simulink model "Clutch_TestBench"  (R2017a)
settings: Solver=FixedStepAuto  StartTime=0.0  StopTime=CycleTime  FixedStep=tloop  RelTol=1e-3
InitFcn:
  | clc
  | clear all;
  | CycleTime=49;
  | tloop=0.01;
undefined symbols (not defined in the file): clt, Clutch, Clutch2, Engine, lib_SystemDiag, SystemDiag
libraries: simulink x23, autolibcoupling x2
settings Model: Creator=Di Russo  LastModifiedBy=Di Russo

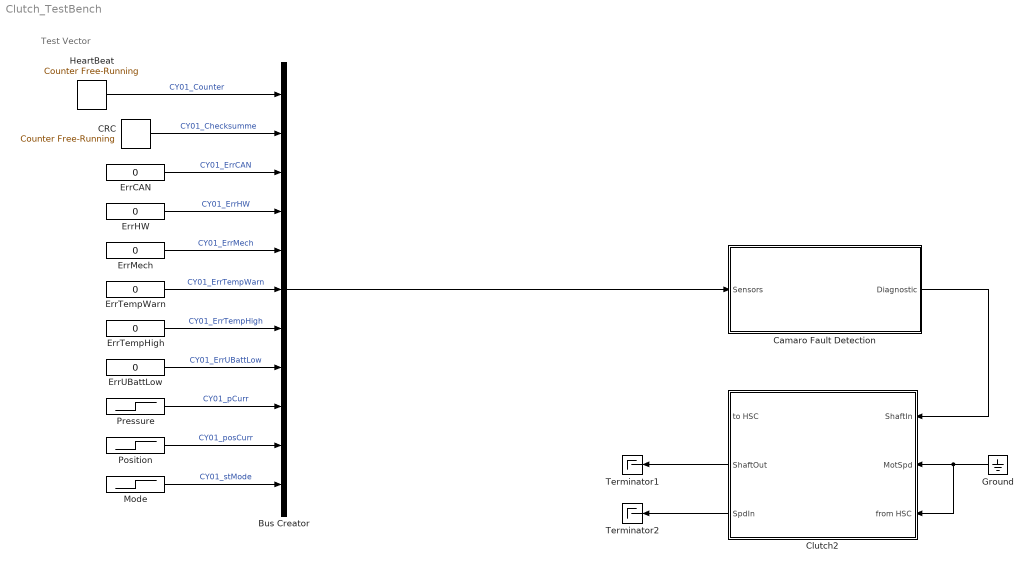
== system Clutch_TestBench ==
  note: Test Vector
  Bus Creator : BusCreator  Inputs=11
  "CRC " : simulink/Sources/Counter Free-Running  NumBits=16  tsamp=-1
  Camaro Fault Detection : Subsystem  AncestorBlock=lib_FaultDetection/Camaro Fault Detection
  Clutch2 : Subsystem  AncestorBlock=Clutch/Clutch2
      mask Display:
      | image('Images/Clutch.jpg')
      | color('red');
      | port_label('Input',1,'From HSC');
      | port_label('Input',2,'ShaftIn');
      | port_label('Input',3,'SpdOut');
      | port_label('Output',1,'To HSC');
      | port_label('Output',2,'ShaftOut');
      | port_label('Output',3,'SpdIn');
  ErrCAN : Constant  Value=0
  ErrHW : Constant  Value=0
  ErrMech : Constant  Value=0
  ErrTempHigh : Constant  Value=0
  ErrTempWarn : Constant  Value=0
  ErrUBattLow : Constant  Value=0
  Ground : Ground
  "HeartBeat " : simulink/Sources/Counter Free-Running  NumBits=4  tsamp=-1
  Mode : Step  After=7  SampleTime=0
  Position : Step  After=7000  SampleTime=0
  Pressure : Step  After=40  SampleTime=0
  Terminator1 : Terminator
  Terminator2 : Terminator
  wires:
  ErrCAN/1 -> Bus Creator/3  "CY01_ErrCAN"
  ErrTempWarn/1 -> Bus Creator/6  "CY01_ErrTempWarn"
  ErrTempHigh/1 -> Bus Creator/7  "CY01_ErrTempHigh"
  ErrUBattLow/1 -> Bus Creator/8  "CY01_ErrUBattLow"
  Pressure/1 -> Bus Creator/9  "CY01_pCurr"
  ErrMech/1 -> Bus Creator/5  "CY01_ErrMech"
  ErrHW/1 -> Bus Creator/4  "CY01_ErrHW"
  Mode/1 -> Bus Creator/11  "CY01_stMode"
  "HeartBeat "/1 -> Bus Creator/1  "CY01_Counter"
  Position/1 -> Bus Creator/10  "CY01_posCurr"
  Bus Creator/1 -> Camaro Fault Detection/1(Sensors)
  "CRC "/1 -> Bus Creator/2  "CY01_Checksumme"
  Camaro Fault Detection/1(Diagnostic) -> Clutch2/1(ShaftIn)
  Ground/1 -> Clutch2/3(from HSC), Clutch2/2(MotSpd)
  Clutch2/2(ShaftOut) -> Terminator1/1
  Clutch2/3(SpdIn) -> Terminator2/1

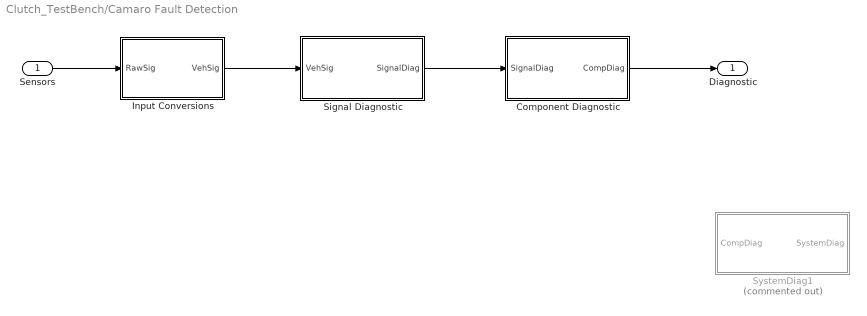
== system Clutch_TestBench/Camaro Fault Detection ==
  Sensors : Inport
  Component Diagnostic : Subsystem
  Input Conversions : Subsystem
  Signal Diagnostic : Subsystem
  SystemDiag1 : Subsystem  Commented=on  AncestorBlock=lib_SystemDiag/SystemDiag
  Diagnostic : Outport
  wires:
  Signal Diagnostic/1(SignalDiag) -> Component Diagnostic/1(SignalDiag)
  Component Diagnostic/1(CompDiag) -> Diagnostic/1
  Input Conversions/1(VehSig) -> Signal Diagnostic/1(VehSig)
  Sensors/1 -> Input Conversions/1(RawSig)

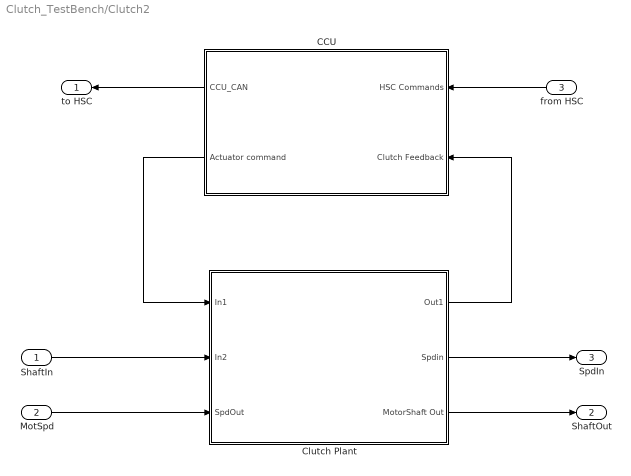
== system Clutch_TestBench/Clutch2 ==
  ShaftIn : Inport
  MotSpd : Inport  Port=2
  from HSC : Inport  Port=3
  CCU : Subsystem
      mask Display: image('SoftECU.jpg')
  Clutch Plant : Subsystem
      mask Display:
      | image('Images/Clutch.jpg')
      | color('red');
      | port_label('Input',2,'ShaftIn');
      | port_label('Input',3,'SpdOut');
      | port_label('Output',3,'ShaftOut');
      | port_label('Output',2,'SpdIn');
  to HSC : Outport
  ShaftOut : Outport  Port=2
  SpdIn : Outport  Port=3
  wires:
  Clutch Plant/1(Out1) -> CCU/2(Clutch Feedback)
  CCU/1("CCU_CAN ") -> to HSC/1
  Clutch Plant/3(MotorShaft Out) -> ShaftOut/1
  Clutch Plant/2(Spdin) -> SpdIn/1
  MotSpd/1 -> Clutch Plant/3(SpdOut)
  ShaftIn/1 -> Clutch Plant/2(In2)
  CCU/2("Actuator command ") -> Clutch Plant/1(In1)
  from HSC/1 -> CCU/1(HSC Commands)

== system Clutch_TestBench/Camaro Fault Detection/Component Diagnostic ==
  note: Component Status Setting Rule
      | xxx_CompStatus could be 0, 1, 2 or 3
      | 0: component needs to be offline
      | 1: component needs torque plant to deliver creep torque
      | 2: component needs torque plant to limit maximum torque delivery
      | 3: component needs torque plant to operate normally
  note: Component Diagnostics
  SignalDiag : Inport
  Clutch Component Diagnostic : Subsystem
  Override Clutch Status : Subsystem
  CompDiag : Outport
  wires:
  Clutch Component Diagnostic/1(Out1) -> Override Clutch Status/1(In1)  "CCM_CompDiag"
  Override Clutch Status/1(Out1) -> CompDiag/1  "Clutch_Status"
  SignalDiag/1 -> Clutch Component Diagnostic/1(In1)  "RawSig"

== system Clutch_TestBench/Camaro Fault Detection/Input Conversions ==
  note: Input Conversions and Override Switches
  note: These subsystems convert variable types to match those used in the
      | supervisor. In addition, override switches installed on each signal can
      | be used to manually override and signal for testing purposes
  RawSig : Inport
  Clutch_Conversions : Subsystem
  VehSig : Outport
  wires:
  Clutch_Conversions/1(Out1) -> VehSig/1
  RawSig/1 -> Clutch_Conversions/1(Sensors)  "RawSig"

== system Clutch_TestBench/Camaro Fault Detection/Signal Diagnostic ==
  note: These subsystems evaluate each signal for proper value range and other checks
  note: Signal Diagnostics
  VehSig : Inport
  Clutch Signal Diagnostic : Subsystem
  Subsystem1 : Subsystem
      mask Display: fprintf('Signal Naming Rule')
  SignalDiag : Outport
  wires:
  Clutch Signal Diagnostic/1(Out2) -> SignalDiag/1  "Clutch_SigDiag"
  VehSig/1 -> Clutch Signal Diagnostic/1(Sensors1)

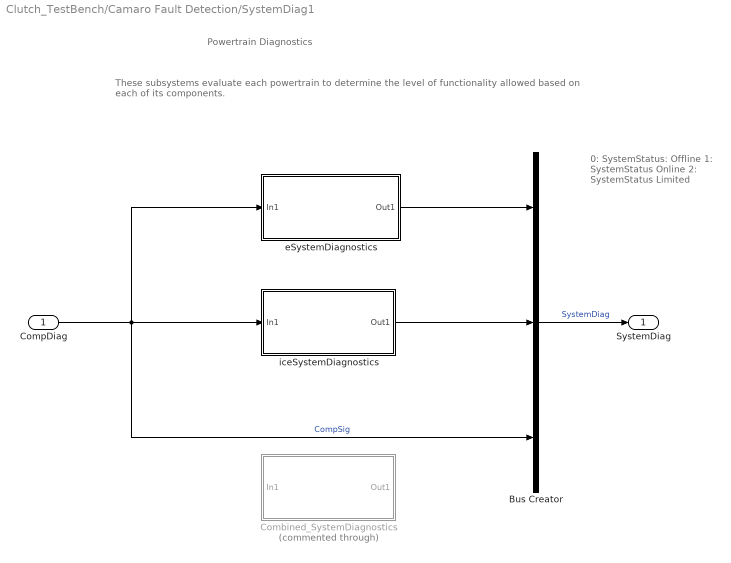
== system Clutch_TestBench/Camaro Fault Detection/SystemDiag1 ==
  note: 0: SystemStatus: Offline
      | 1: SystemStatus Online
      | 2: SystemStatus Limited
  note: Powertrain Diagnostics
  note: These subsystems evaluate each powertrain to determine
      | the level of functionality allowed based on each of its components.
  CompDiag : Inport
  Bus Creator : BusCreator  Inputs=3
  Combined_SystemDiagnostics : Subsystem  Commented=through
  eSystemDiagnostics : Subsystem
  iceSystemDiagnostics : Subsystem
  SystemDiag : Outport
  wires:
  eSystemDiagnostics/1(Out1) -> Bus Creator/1
  Bus Creator/1 -> SystemDiag/1  "SystemDiag"
  CompDiag/1 -> iceSystemDiagnostics/1(In1), Bus Creator/3, eSystemDiagnostics/1(In1)  "CompSig"
  iceSystemDiagnostics/1(Out1) -> Bus Creator/2

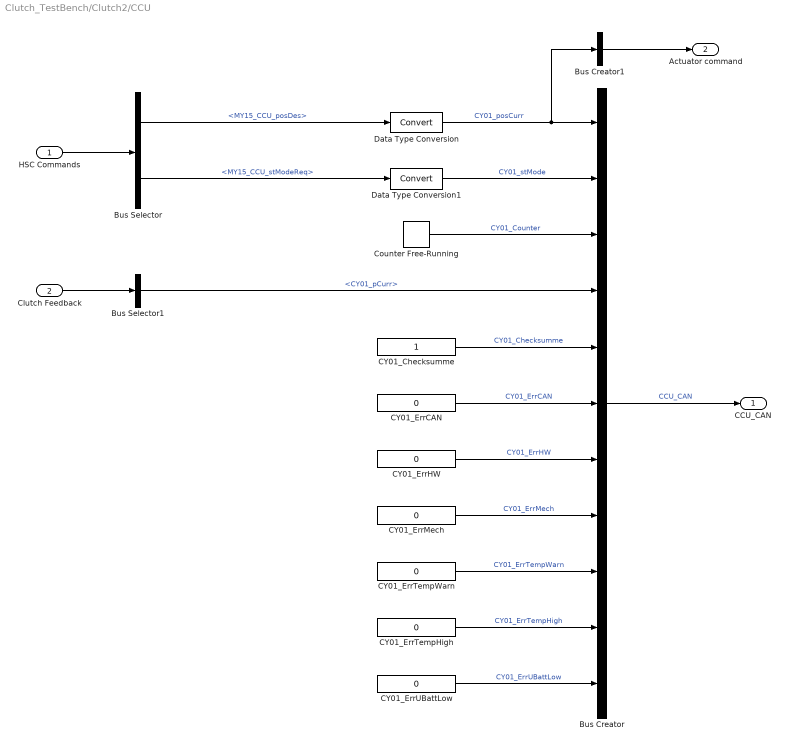
== system Clutch_TestBench/Clutch2/CCU ==
  HSC Commands : Inport
  Clutch Feedback : Inport  Port=2
  Bus Creator : BusCreator  Inputs=11
  Bus Creator1 : BusCreator  Inputs=1
  Bus Selector : BusSelector  OutputSignals=MY15_CCU_posDes,MY15_CCU_stModeReq
  Bus Selector1 : BusSelector  OutputSignals=CY01_pCurr
  CY01_Checksumme : Constant
  CY01_ErrCAN : Constant  Value=0
  CY01_ErrHW : Constant  Value=0
  CY01_ErrMech : Constant  Value=0
  CY01_ErrTempHigh : Constant  Value=0
  CY01_ErrTempWarn : Constant  Value=0
  CY01_ErrUBattLow : Constant  Value=0
  Counter Free-Running : simulink/Sources/Counter Free-Running  NumBits=15  tsamp=-1
  Data Type Conversion : DataTypeConversion
  Data Type Conversion1 : DataTypeConversion
  "CCU_CAN " : Outport
  "Actuator command " : Outport  Port=2
  wires:
  Clutch Feedback/1 -> Bus Selector1/1
  Data Type Conversion1/1 -> Bus Creator/2  "CY01_stMode"
  Bus Selector/2 -> Data Type Conversion1/1  "<MY15_CCU_stModeReq>"
  Counter Free-Running/1 -> Bus Creator/3  "CY01_Counter"
  Bus Creator1/1 -> "Actuator command "/1
  Bus Creator/1 -> "CCU_CAN "/1  "CCU_CAN"
  Data Type Conversion/1 -> Bus Creator1/1, Bus Creator/1  "CY01_posCurr"
  Bus Selector/1 -> Data Type Conversion/1  "<MY15_CCU_posDes>"
  HSC Commands/1 -> Bus Selector/1
  Bus Selector1/1 -> Bus Creator/4  "<CY01_pCurr>"
  CY01_Checksumme/1 -> Bus Creator/5  "CY01_Checksumme"
  CY01_ErrCAN/1 -> Bus Creator/6  "CY01_ErrCAN"
  CY01_ErrHW/1 -> Bus Creator/7  "CY01_ErrHW"
  CY01_ErrMech/1 -> Bus Creator/8  "CY01_ErrMech"
  CY01_ErrUBattLow/1 -> Bus Creator/11  "CY01_ErrUBattLow"
  CY01_ErrTempHigh/1 -> Bus Creator/10  "CY01_ErrTempHigh"
  CY01_ErrTempWarn/1 -> Bus Creator/9  "CY01_ErrTempWarn"

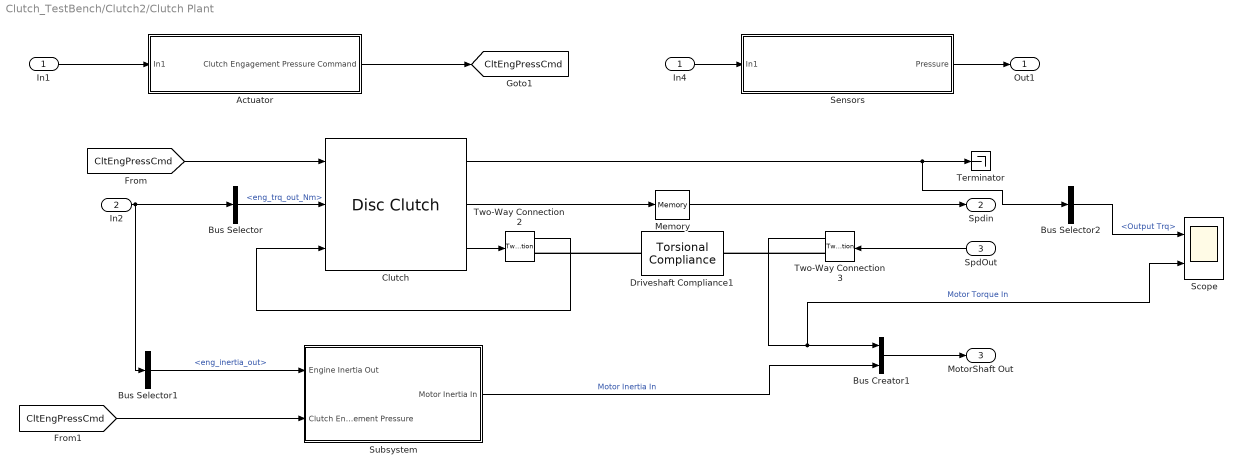
== system Clutch_TestBench/Clutch2/Clutch Plant ==
  In1 : Inport
  In2 : Inport  Port=2
  SpdOut : Inport  Port=3
  " Actuator" : Subsystem
  " Sensors " : Subsystem
  Bus Creator1 : BusCreator  Inputs=2
  Bus Selector : BusSelector  OutputSignals=eng_trq_out_Nm
  Bus Selector1 : BusSelector  OutputSignals=eng_inertia_out
  Bus Selector2 : BusSelector  OutputSignals=Output.Output Trq
  Clutch : autolibcoupling/Disc Clutch  port_config=Simulink  Reff=0.121  Ndisk=1  Aeff=0.02129  Jin=Engine.Inertia + (0.75*clt.plant.init.inertia)  Jout=.1 + (0.25*clt.plant.init.inertia)  muk=0.25  mus=0.3  bin=.001*2  bout=.001*2  win_o=0  wout_o=0  tauC=0.01*10  InitiallyLocked=on  maxAbsSpd=3000  blkID=1
      settings: SourceProductName=Powertrain Blockset  SourceProductBaseCode=PW
  Driveshaft Compliance1 : autolibcoupling/Torsional Compliance  port_config=Two-way connection  k=1000000  b=100  theta_o=0  domega_o=0  omega_c=100  blkID=0
      settings: SourceProductName=Powertrain Blockset
  In4 : InportShadow
  Memory : Memory
  Scope : Scope  NumInputPorts=2
  Subsystem : Subsystem
  Terminator : Terminator
  Two-Way Connection2 : TwoWayConnection
  Two-Way Connection3 : TwoWayConnection
  Out1 : Outport
  Spdin : Outport  Port=2
  MotorShaft Out : Outport  Port=3
  tag scope: CltEngPressCmd=global
  wires:
  " Sensors "/1(Pressure) -> Out1/1
  In4/1 -> " Sensors "/1(In1)
  Bus Selector/1 -> Clutch/2  "<eng_trq_out_Nm>"
  [CltEngPressCmd] -> Clutch/1
  " Actuator"/1(Clutch Engagement Pressure Command) -> [CltEngPressCmd]
  Clutch/1 -> Bus Selector2/1, Terminator/1
  In1/1 -> " Actuator"/1(In1)
  Clutch/3 -> Two-Way Connection2/1
  SpdOut/1 -> Two-Way Connection3/1
  In2/1 -> Bus Selector1/1, Bus Selector/1
  Memory/1 -> Spdin/1
  Two-Way Connection2/1 -> Clutch/3
  Two-Way Connection3/1 -> Scope/2, Bus Creator1/1  "Motor Torque In"
  Clutch/2 -> Memory/1
  [CltEngPressCmd] -> Subsystem/2(Clutch Engagement Pressure)
  Bus Selector1/1 -> Subsystem/1(Engine Inertia Out)  "<eng_inertia_out>"
  Bus Creator1/1 -> MotorShaft Out/1
  Subsystem/1(Motor Inertia In) -> Bus Creator1/2  "Motor Inertia In"
  Bus Selector2/1 -> Scope/1  "<Output Trq>"
  connections:
  Driveshaft Compliance1/LConn1 -- Two-Way Connection2/RConn1
  Two-Way Connection3/RConn1 -- Driveshaft Compliance1/RConn1

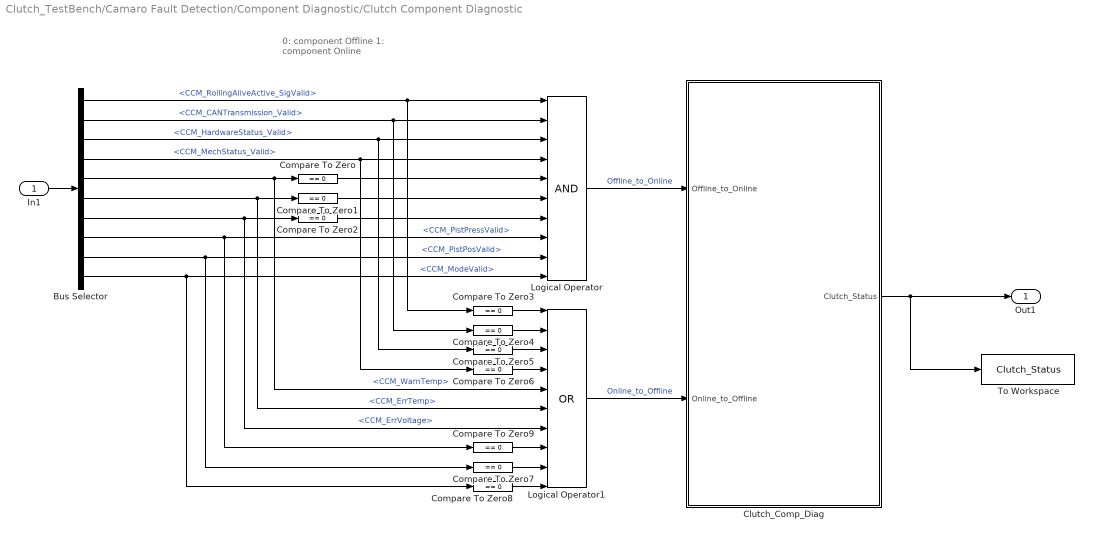
== system Clutch_TestBench/Camaro Fault Detection/Component Diagnostic/Clutch Component Diagnostic ==
  note: 0: component Offline
      | 1: component Online
  In1 : Inport
  Bus Selector : BusSelector  OutputSignals=CCM_RollingAliveActive_SigValid,CCM_CANTransmission_Valid,CCM_HardwareStatus_Valid,CCM_MechStatus_Valid,CCM_WarnTemp,CCM_ErrTemp,CCM_ErrVoltage,CCM_PistPressValid,CCM_PistPosValid,CCM_ModeValid
  Clutch_Comp_Diag : Stateflow chart  TreatAsAtomicUnit=on
  Compare To Zero{,1..9} (10 alike) : simulink/Logic and Bit Operations/Compare To Zero  relop===  OutDataTypeStr=boolean
  Logical Operator : Logic  Inputs=10  AllPortsSameDT=off  OutDataTypeStr=boolean
  Logical Operator1 : Logic  Operator=OR  Inputs=10  AllPortsSameDT=off  OutDataTypeStr=boolean
  To Workspace : ToWorkspace  VariableName=Clutch_Status  SampleTime=-1
  Out1 : Outport
  wires:
  In1/1 -> Bus Selector/1
  Bus Selector/1 -> Compare To Zero3/1, Logical Operator/1  "<CCM_RollingAliveActive_SigValid>"
  Bus Selector/2 -> Compare To Zero4/1, Logical Operator/2  "<CCM_CANTransmission_Valid>"
  Bus Selector/3 -> Compare To Zero5/1, Logical Operator/3  "<CCM_HardwareStatus_Valid>"
  Bus Selector/4 -> Compare To Zero6/1, Logical Operator/4  "<CCM_MechStatus_Valid>"
  Bus Selector/5 -> Logical Operator1/5, Compare To Zero/1  "<CCM_WarnTemp>"
  Bus Selector/6 -> Logical Operator1/6, Compare To Zero1/1  "<CCM_ErrTemp>"
  Bus Selector/7 -> Logical Operator1/7, Compare To Zero2/1  "<CCM_ErrVoltage>"
  Bus Selector/8 -> Compare To Zero9/1, Logical Operator/8  "<CCM_PistPressValid>"
  Bus Selector/9 -> Compare To Zero7/1, Logical Operator/9  "<CCM_PistPosValid>"
  Bus Selector/10 -> Compare To Zero8/1, Logical Operator/10  "<CCM_ModeValid>"
  Logical Operator/1 -> Clutch_Comp_Diag/1(Offline_to_Online)  "Offline_to_Online"
  Logical Operator1/1 -> Clutch_Comp_Diag/2(Online_to_Offline)  "Online_to_Offline"
  Clutch_Comp_Diag/1(Clutch_Status) -> To Workspace/1, Out1/1
  Compare To Zero/1 -> Logical Operator/5
  Compare To Zero1/1 -> Logical Operator/6
  Compare To Zero2/1 -> Logical Operator/7
  Compare To Zero3/1 -> Logical Operator1/1
  Compare To Zero4/1 -> Logical Operator1/2
  Compare To Zero5/1 -> Logical Operator1/3
  Compare To Zero6/1 -> Logical Operator1/4
  Compare To Zero7/1 -> Logical Operator1/9
  Compare To Zero8/1 -> Logical Operator1/10
  Compare To Zero9/1 -> Logical Operator1/8

== system Clutch_TestBench/Camaro Fault Detection/Component Diagnostic/Override Clutch Status ==
  note: This subsystem is used to override the model value of a signal to a constant value
  note: Override Switch Subsystem
  In1 : Inport
  Multiport Switch : MultiPortSwitch  DataPortOrder=Zero-based contiguous  Inputs=2  zeroidx=on
  Override Value : Constant  Value=2  OutDataTypeStr=double
  Signal Override Switch 0 = Use Model 1 = Use Constant : Constant  Value=0
  Out1 : Outport
  wires:
  Signal Override Switch 0 = Use Model 1 = Use Constant/1 -> Multiport Switch/1
  In1/1 -> Multiport Switch/2
  Multiport Switch/1 -> Out1/1
  Override Value/1 -> Multiport Switch/3

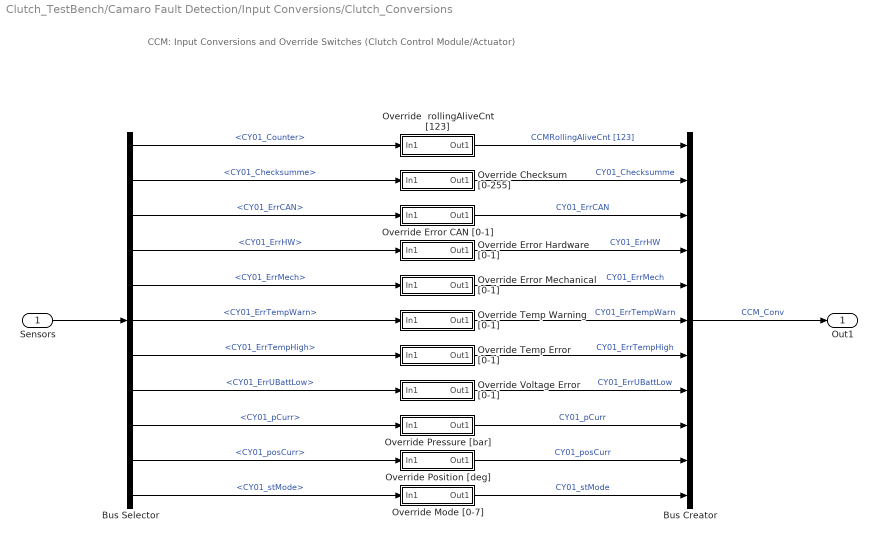
== system Clutch_TestBench/Camaro Fault Detection/Input Conversions/Clutch_Conversions ==
  note: CCM: Input Conversions and Override Switches
      | (Clutch Control Module/Actuator)
  Sensors : Inport
  Bus Creator : BusCreator  Inputs=11
  Bus Selector : BusSelector  OutputSignals=CY01_Counter,CY01_Checksumme,CY01_ErrCAN,CY01_ErrHW,CY01_ErrMech,CY01_ErrTempWarn,CY01_ErrTempHigh,CY01_ErrUBattLow,CY01_pCurr,CY01_posCurr,CY01_stMode
  Override  rollingAliveCnt [123] : Subsystem
  Override Checksum [0-255] : Subsystem
  Override Error CAN [0-1] : Subsystem
  Override Error Hardware [0-1] : Subsystem
  Override Error Mechanical [0-1] : Subsystem
  Override Mode [0-7] : Subsystem
  Override Position [deg] : Subsystem
  Override Pressure [bar] : Subsystem
  Override Temp Error [0-1] : Subsystem
  Override Temp Warning [0-1] : Subsystem
  Override Voltage Error [0-1] : Subsystem
  Out1 : Outport
  wires:
  Override Mode [0-7]/1(Out1) -> Bus Creator/11  "CY01_stMode"
  Override Position [deg]/1(Out1) -> Bus Creator/10  "CY01_posCurr"
  Override Pressure [bar]/1(Out1) -> Bus Creator/9  "CY01_pCurr"
  Bus Selector/11 -> Override Mode [0-7]/1(In1)  "<CY01_stMode>"
  Bus Selector/10 -> Override Position [deg]/1(In1)  "<CY01_posCurr>"
  Bus Selector/9 -> Override Pressure [bar]/1(In1)  "<CY01_pCurr>"
  Override Voltage Error [0-1]/1(Out1) -> Bus Creator/8  "CY01_ErrUBattLow"
  Override Temp Error [0-1]/1(Out1) -> Bus Creator/7  "CY01_ErrTempHigh"
  Override Temp Warning [0-1]/1(Out1) -> Bus Creator/6  "CY01_ErrTempWarn"
  Override Error Mechanical [0-1]/1(Out1) -> Bus Creator/5  "CY01_ErrMech"
  Override Error Hardware [0-1]/1(Out1) -> Bus Creator/4  "CY01_ErrHW"
  Override Error CAN [0-1]/1(Out1) -> Bus Creator/3  "CY01_ErrCAN"
  Override Checksum [0-255]/1(Out1) -> Bus Creator/2  "CY01_Checksumme"
  Bus Selector/8 -> Override Voltage Error [0-1]/1(In1)  "<CY01_ErrUBattLow>"
  Bus Selector/7 -> Override Temp Error [0-1]/1(In1)  "<CY01_ErrTempHigh>"
  Bus Selector/6 -> Override Temp Warning [0-1]/1(In1)  "<CY01_ErrTempWarn>"
  Bus Selector/5 -> Override Error Mechanical [0-1]/1(In1)  "<CY01_ErrMech>"
  Bus Selector/4 -> Override Error Hardware [0-1]/1(In1)  "<CY01_ErrHW>"
  Bus Selector/3 -> Override Error CAN [0-1]/1(In1)  "<CY01_ErrCAN>"
  Bus Selector/2 -> Override Checksum [0-255]/1(In1)  "<CY01_Checksumme>"
  Sensors/1 -> Bus Selector/1
  Bus Selector/1 -> Override  rollingAliveCnt [123]/1(In1)  "<CY01_Counter>"
  Override  rollingAliveCnt [123]/1(Out1) -> Bus Creator/1  "CCMRollingAliveCnt [123]"
  Bus Creator/1 -> Out1/1  "CCM_Conv"

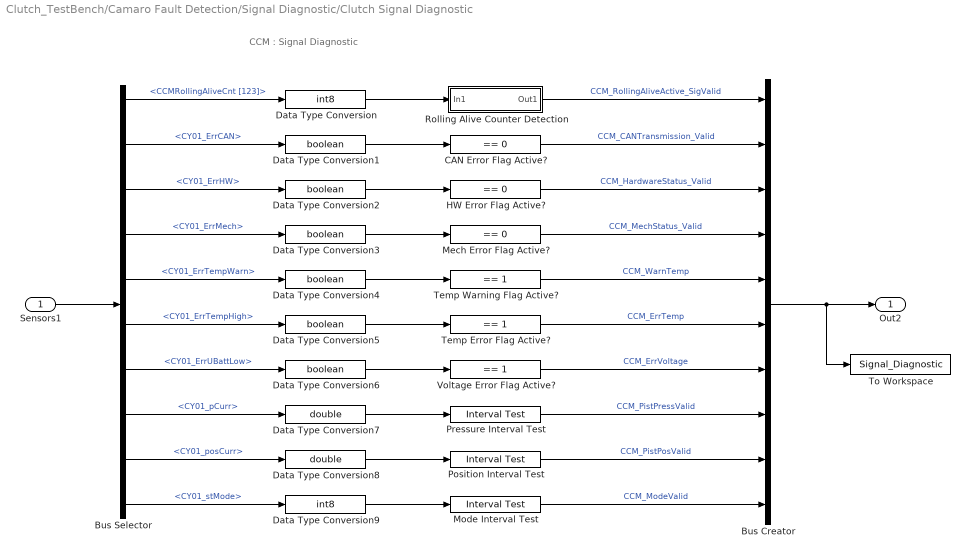
== system Clutch_TestBench/Camaro Fault Detection/Signal Diagnostic/Clutch Signal Diagnostic ==
  note: CCM : Signal Diagnostic
  Sensors1 : Inport
  Bus Creator : BusCreator  Inputs=10
  Bus Selector : BusSelector  OutputSignals=CCMRollingAliveCnt [123],CY01_ErrCAN,CY01_ErrHW,CY01_ErrMech,CY01_ErrTempWarn,CY01_ErrTempHigh,CY01_ErrUBattLow,CY01_pCurr,CY01_posCurr,CY01_stMode
  CAN Error Flag Active? : simulink/Logic and Bit Operations/Compare To Constant  relop===  const=0  OutDataTypeStr=boolean
  Data Type Conversion : DataTypeConversion  OutDataTypeStr=int8
  Data Type Conversion{1..6} (6 alike) : DataTypeConversion  OutDataTypeStr=boolean
  Data Type Conversion7 : DataTypeConversion  OutDataTypeStr=double
  Data Type Conversion8 : DataTypeConversion  OutDataTypeStr=double
  Data Type Conversion9 : DataTypeConversion  OutDataTypeStr=int8
  HW Error Flag Active? : simulink/Logic and Bit Operations/Compare To Constant  relop===  const=0  OutDataTypeStr=boolean
  Mech Error Flag Active? : simulink/Logic and Bit Operations/Compare To Constant  relop===  const=0  OutDataTypeStr=boolean
  Mode Interval Test : simulink/Logic and Bit Operations/Interval Test  IntervalClosedRight=on  uplimit=7  IntervalClosedLeft=on  lowlimit=0  OutDataTypeStr=boolean
  Position Interval Test : simulink/Logic and Bit Operations/Interval Test  IntervalClosedRight=on  uplimit=8190  IntervalClosedLeft=on  lowlimit=0  OutDataTypeStr=boolean
  Pressure Interval Test : simulink/Logic and Bit Operations/Interval Test  IntervalClosedRight=on  uplimit=50.6  IntervalClosedLeft=on  lowlimit=0  OutDataTypeStr=boolean
  Rolling Alive Counter Detection : Subsystem
  Temp Error Flag Active? : simulink/Logic and Bit Operations/Compare To Constant  relop===  const=1  OutDataTypeStr=boolean
  Temp Warning Flag Active? : simulink/Logic and Bit Operations/Compare To Constant  relop===  const=1  OutDataTypeStr=boolean
  To Workspace : ToWorkspace  VariableName=Signal_Diagnostic  SampleTime=-1
  Voltage Error Flag Active? : simulink/Logic and Bit Operations/Compare To Constant  relop===  const=1  OutDataTypeStr=boolean
  Out2 : Outport
  wires:
  Mode Interval Test/1 -> Bus Creator/10  "CCM_ModeValid"
  Bus Selector/10 -> Data Type Conversion9/1  "<CY01_stMode>"
  Position Interval Test/1 -> Bus Creator/9  "CCM_PistPosValid"
  Bus Selector/9 -> Data Type Conversion8/1  "<CY01_posCurr>"
  Pressure Interval Test/1 -> Bus Creator/8  "CCM_PistPressValid"
  Bus Selector/8 -> Data Type Conversion7/1  "<CY01_pCurr>"
  Voltage Error Flag Active?/1 -> Bus Creator/7  "CCM_ErrVoltage"
  Bus Selector/7 -> Data Type Conversion6/1  "<CY01_ErrUBattLow>"
  Temp Error Flag Active?/1 -> Bus Creator/6  "CCM_ErrTemp"
  Bus Selector/6 -> Data Type Conversion5/1  "<CY01_ErrTempHigh>"
  Temp Warning Flag Active?/1 -> Bus Creator/5  "CCM_WarnTemp"
  Bus Selector/5 -> Data Type Conversion4/1  "<CY01_ErrTempWarn>"
  Mech Error Flag Active?/1 -> Bus Creator/4  "CCM_MechStatus_Valid"
  Bus Selector/4 -> Data Type Conversion3/1  "<CY01_ErrMech>"
  HW Error Flag Active?/1 -> Bus Creator/3  "CCM_HardwareStatus_Valid"
  Bus Selector/3 -> Data Type Conversion2/1  "<CY01_ErrHW>"
  CAN Error Flag Active?/1 -> Bus Creator/2  "CCM_CANTransmission_Valid"
  Bus Selector/2 -> Data Type Conversion1/1  "<CY01_ErrCAN>"
  Rolling Alive Counter Detection/1(Out1) -> Bus Creator/1  "CCM_RollingAliveActive_SigValid"
  Bus Selector/1 -> Data Type Conversion/1  "<CCMRollingAliveCnt [123]>"
  Bus Creator/1 -> To Workspace/1, Out2/1
  Sensors1/1 -> Bus Selector/1
  Data Type Conversion/1 -> Rolling Alive Counter Detection/1(In1)
  Data Type Conversion1/1 -> CAN Error Flag Active?/1
  Data Type Conversion2/1 -> HW Error Flag Active?/1
  Data Type Conversion3/1 -> Mech Error Flag Active?/1
  Data Type Conversion4/1 -> Temp Warning Flag Active?/1
  Data Type Conversion5/1 -> Temp Error Flag Active?/1
  Data Type Conversion6/1 -> Voltage Error Flag Active?/1
  Data Type Conversion7/1 -> Pressure Interval Test/1
  Data Type Conversion8/1 -> Position Interval Test/1
  Data Type Conversion9/1 -> Mode Interval Test/1

== system Clutch_TestBench/Camaro Fault Detection/Signal Diagnostic/Subsystem1 ==
  note: Signal Valid Setting Rule
      | xxx_yyy_[z]_SigValid could be 0 or 1
      | 0: signal invalid
      | 1: signal vaild
  note: Signal Naming Rule
      | Example: xxx_yyy_[z]_SigValid
      | xxx: source of the signal (Drv, Clu, BCM, ECM, TCM, BMS and MCU)
      | yyy: description of the signal
      | z: unit of the signal (V, A, Nm, m/s, %, 01, 0123, etc.)

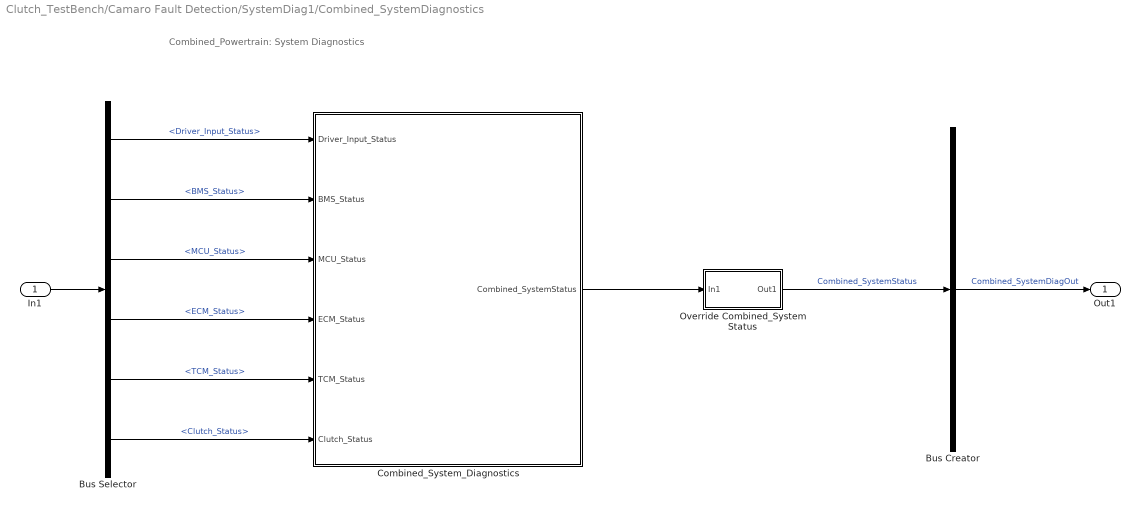
== system Clutch_TestBench/Camaro Fault Detection/SystemDiag1/Combined_SystemDiagnostics ==
  note: Combined_Powertrain: System Diagnostics
  In1 : Inport
  Bus Creator : BusCreator  Inputs=1
  Bus Selector : BusSelector  OutputSignals=Driver_Input_Status.Driver_Input_Status,BMS_Status.BMS_Status,MCU_Status.MCU_Status,ECM_Status.ECM_Status,TCM_CompDiag.TCM_Status,Clutch_Status.Clutch_Status
  Combined_System_Diagnostics : Stateflow chart  TreatAsAtomicUnit=on
  Override Combined_System Status : Subsystem
  Out1 : Outport
  wires:
  In1/1 -> Bus Selector/1
  Bus Creator/1 -> Out1/1  "Combined_SystemDiagOut"
  Override Combined_System Status/1(Out1) -> Bus Creator/1  "Combined_SystemStatus"
  Bus Selector/1 -> Combined_System_Diagnostics/1(Driver_Input_Status)  "<Driver_Input_Status>"
  Bus Selector/2 -> Combined_System_Diagnostics/2(BMS_Status)  "<BMS_Status>"
  Bus Selector/3 -> Combined_System_Diagnostics/3(MCU_Status)  "<MCU_Status>"
  Bus Selector/4 -> Combined_System_Diagnostics/4(ECM_Status)  "<ECM_Status>"
  Bus Selector/5 -> Combined_System_Diagnostics/5(TCM_Status)  "<TCM_Status>"
  Bus Selector/6 -> Combined_System_Diagnostics/6(Clutch_Status)  "<Clutch_Status>"
  Combined_System_Diagnostics/1(Combined_SystemStatus) -> Override Combined_System Status/1(In1)

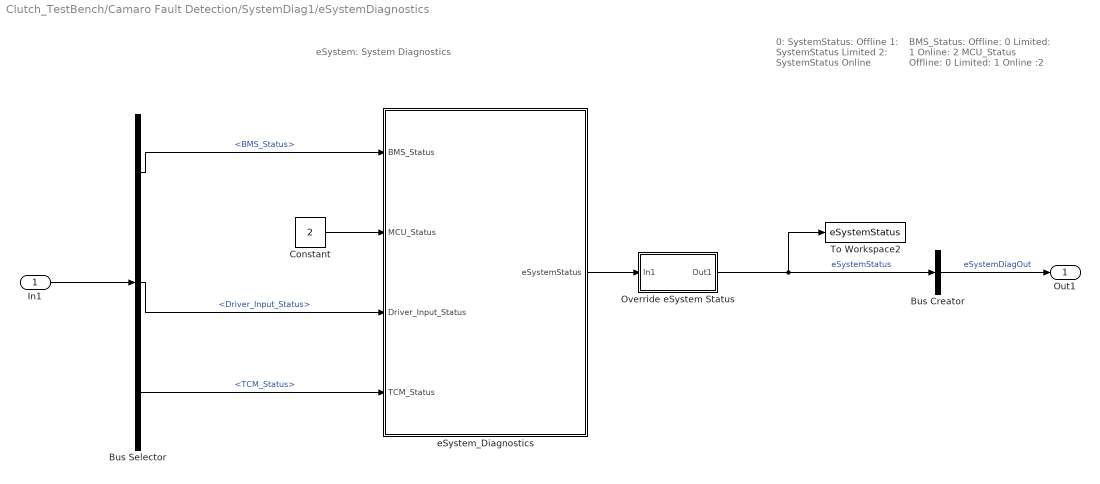
== system Clutch_TestBench/Camaro Fault Detection/SystemDiag1/eSystemDiagnostics ==
  note: BMS_Status:
      | Offline: 0
      | Limited: 1
      | Online: 2
      |
      | MCU_Status
      | Offline: 0
      | Limited: 1
      | Online :2
  note: 0: SystemStatus: Offline
      | 1: SystemStatus Limited
      | 2: SystemStatus Online
  note: eSystem: System Diagnostics
  In1 : Inport
  Bus Creator : BusCreator  Inputs=1
  Bus Selector : BusSelector  OutputSignals=BMS_Status,Driver_Input_Status,TCM_Status
  Constant : Constant  Value=2
  Override eSystem Status : Subsystem
  To Workspace2 : ToWorkspace  VariableName=eSystemStatus  SaveFormat=Timeseries  SampleTime=-1
  eSystem_Diagnostics : Stateflow chart  TreatAsAtomicUnit=on
  Out1 : Outport
  wires:
  Constant/1 -> eSystem_Diagnostics/2(MCU_Status)
  In1/1 -> Bus Selector/1
  Bus Selector/1 -> eSystem_Diagnostics/1(BMS_Status)  "<BMS_Status>"
  Bus Creator/1 -> Out1/1  "eSystemDiagOut"
  Bus Selector/2 -> eSystem_Diagnostics/3(Driver_Input_Status)  "<Driver_Input_Status>"
  Override eSystem Status/1(Out1) -> To Workspace2/1, Bus Creator/1  "eSystemStatus"
  eSystem_Diagnostics/1(eSystemStatus) -> Override eSystem Status/1(In1)
  Bus Selector/3 -> eSystem_Diagnostics/4(TCM_Status)  "<TCM_Status>"

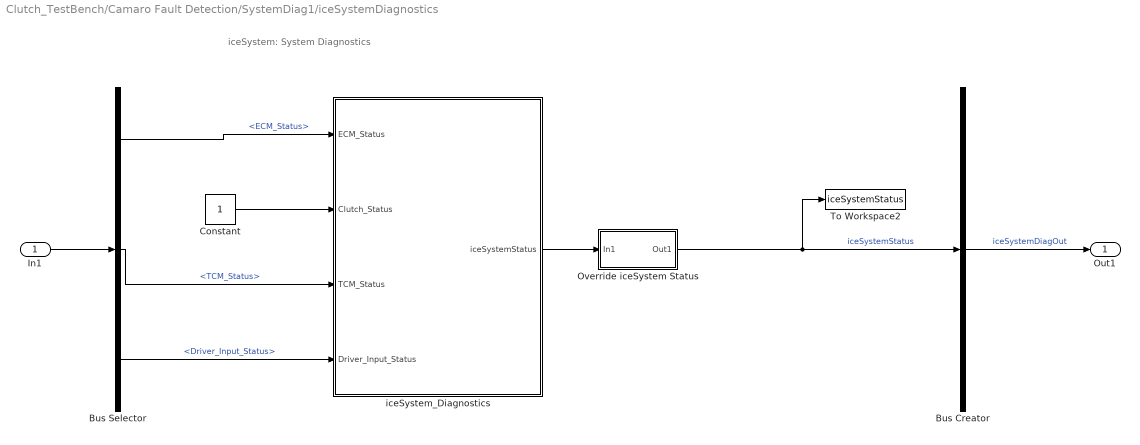
== system Clutch_TestBench/Camaro Fault Detection/SystemDiag1/iceSystemDiagnostics ==
  note: iceSystem: System Diagnostics
  In1 : Inport
  Bus Creator : BusCreator  Inputs=1
  Bus Selector : BusSelector  OutputSignals=ECM_Status,TCM_Status,Driver_Input_Status
  Constant : Constant
  Override iceSystem Status : Subsystem
  To Workspace2 : ToWorkspace  VariableName=iceSystemStatus  SaveFormat=Timeseries  SampleTime=-1
  iceSystem_Diagnostics : Stateflow chart  TreatAsAtomicUnit=on
  Out1 : Outport
  wires:
  Override iceSystem Status/1(Out1) -> To Workspace2/1, Bus Creator/1  "iceSystemStatus"
  Bus Selector/1 -> iceSystem_Diagnostics/1(ECM_Status)  "<ECM_Status>"
  Bus Creator/1 -> Out1/1  "iceSystemDiagOut"
  In1/1 -> Bus Selector/1
  Bus Selector/2 -> iceSystem_Diagnostics/3(TCM_Status)  "<TCM_Status>"
  Bus Selector/3 -> iceSystem_Diagnostics/4(Driver_Input_Status)  "<Driver_Input_Status>"
  iceSystem_Diagnostics/1(iceSystemStatus) -> Override iceSystem Status/1(In1)
  Constant/1 -> iceSystem_Diagnostics/2(Clutch_Status)

== system Clutch_TestBench/Clutch2/Clutch Plant/ Actuator ==
  In1 : Inport
  Actuator Position to Clutch Engagement Pressure : Lookup_n-D  NumberOfTableDimensions=1  BreakpointsForDimension1=|  Table=|  InternalRulePriority=Speed  RndMeth=Simplest  InputSameDT=on
      BreakpointsForDimension1=|
      | [0
      | 100
      | 200
      | 300
      | 400
      | 500
      | 600
      | 700
      | 800
      | 900
      | 1000
      | 1100
      | 1200
      | 1300
      | 1400
      | 1500
      | 1600
      | 1700
      | 1800
      | 1900
      | 2000
      | 2100
      | 2200
      | 2300
      | 2400
      | 2500
      | 2600
      | 2700
      | 2800
      | 2900
      | 3000
      | 3100
      | 3200
      | 3300
      | 3400
      | 3500
      | 3600
      | 3700
      | 3800
      | 3900
      | 4000
      | 4100
      | 4200
      | 4300
      | 4400
      | 4500
      | 4600
      | 4700
      | 4800
      | 4900
      | 5000
      | 5100
      | 5200
      | 5300
      | 5400
      | 5500
      | 5600
      | 5700
      | 5800
      | 5900
      | 6000
      | 6100
      | 6200
      | 6300
      | 6400
      | 
      | ]
      Table=|
      | [892800
      | 892800
      | 892800
      | 833280
      | 773760
      | 714240
      | 654720
      | 595200
      | 535680
      | 476160
      | 416640
      | 357120
      | 297600
      | 238080
      | 178560
      | 119040
      | 59520
      | 0
      | 0
      | 0
      | 0
      | 0
      | 0
      | 0
      | 0
      | 0
      | 0
      | 0
      | 0
      | 0
      | 0
      | 0
      | 0
      | 0
      | 0
      | 0
      | 0
      | 0
      | 0
      | 0
      | 0
      | 0
      | 0
      | 0
      | 0
      | 0
      | 0
      | 0
      | 0
      | 0
      | 0
      | 0
      | 0
      | 0
      | 0
      | 0
      | 0
      | 0
      | 0
      | 0
      | 0
      | 0
      | 0
      | 0
      | 0
      | 
      | 
      | ]
  Bus Selector : BusSelector  OutputSignals=CY01_posCurr
  Clutch Engagement Pressure Command : Outport
  wires:
  Actuator Position to Clutch Engagement Pressure/1 -> Clutch Engagement Pressure Command/1
  Bus Selector/1 -> Actuator Position to Clutch Engagement Pressure/1  "<CY01_posCurr>"
  In1/1 -> Bus Selector/1

== system Clutch_TestBench/Clutch2/Clutch Plant/ Sensors  ==
  In1 : Inport
  Actuator Position to Actuator Pressure : Lookup_n-D  NumberOfTableDimensions=1  BreakpointsForDimension1=|  Table=|  InternalRulePriority=Speed  RndMeth=Simplest  InputSameDT=on
      BreakpointsForDimension1=|
      | [0
      | 300
      | 400
      | 500
      | 600
      | 700
      | 800
      | 900
      | 1000
      | 1100
      | 1200
      | 1300
      | 1400
      | 1500
      | 1600
      | 1700
      | 1800
      | 1900
      | 2000
      | 2100
      | 2200
      | 2300
      | 2400
      | 2500
      | 2600
      | 2700
      | 2800
      | 2900
      | 3000
      | 3100
      | 3200
      | 3300
      | 3400
      | 3500
      | 3600
      | 3700
      | 3800
      | 3900
      | 4000
      | 4100
      | 4200
      | 4300
      | 4400
      | 4500
      | 4600
      | 4650
      | ]
      Table=|
      | [0.4
      | 1.2
      | 2.6
      | 4
      | 5.6
      | 6.8
      | 8.6
      | 10.4
      | 12.2
      | 14
      | 15.8
      | 17.4
      | 18.8
      | 19.6
      | 20.2
      | 20
      | 19.8
      | 19.6
      | 19
      | 18.8
      | 18.4
      | 18
      | 17.8
      | 17.6
      | 17.4
      | 17.2
      | 17
      | 16.8
      | 16.6
      | 16.6
      | 16.6
      | 16.8
      | 17
      | 17.2
      | 17.4
      | 17.8
      | 18
      | 18.4
      | 18.6
      | 19
      | 19.4
      | 20.4
      | 21.2
      | 25.4
      | 36.4
      | 41
      | ]
  Bus Creator : BusCreator  Inputs=1
  Bus Selector : BusSelector  OutputSignals=CY01_posCurr
  Pressure : Outport
  wires:
  Bus Creator/1 -> Pressure/1
  In1/1 -> Bus Selector/1
  Bus Selector/1 -> Actuator Position to Actuator Pressure/1  "<CY01_posCurr>"
  Actuator Position to Actuator Pressure/1 -> Bus Creator/1  "CY01_pCurr"

== system Clutch_TestBench/Clutch2/Clutch Plant/Subsystem ==
  Engine Inertia Out : Inport
  Clutch Engagement Pressure : Inport  Port=2
  Clutch Inertia : Constant  Value=clt.plant.init.inertia
  Sum5 : Sum  Inputs=++|  SaturateOnIntegerOverflow=on  InputSameDT=on  OutDataTypeStr=Inherit: Same as first input
  Switch2 : Switch  Criteria=u2 > Threshold  SaturateOnIntegerOverflow=on  InputSameDT=on
  Motor Inertia In : Outport
  wires:
  Switch2/1 -> Motor Inertia In/1
  Engine Inertia Out/1 -> Sum5/2
  Sum5/1 -> Switch2/1
  Clutch Inertia/1 -> Switch2/3, Sum5/1
  Clutch Engagement Pressure/1 -> Switch2/2

== system Clutch_TestBench/Camaro Fault Detection/Input Conversions/Clutch_Conversions/Override  rollingAliveCnt [123] ==
  note: Override Switch Subsystem
  note: This subsystem is used to override the model value of a signal to a constant value
  In1 : Inport
  Multiport Switch : MultiPortSwitch  DataPortOrder=Zero-based contiguous  Inputs=2  zeroidx=on
  Override Value : Constant  Value=0  OutDataTypeStr=double
  Signal Override Switch 0 = Use Model 1 = Use Constant : Constant  Value=0
  Out1 : Outport
  wires:
  Override Value/1 -> Multiport Switch/3
  Multiport Switch/1 -> Out1/1
  In1/1 -> Multiport Switch/2
  Signal Override Switch 0 = Use Model 1 = Use Constant/1 -> Multiport Switch/1

== system Clutch_TestBench/Camaro Fault Detection/Input Conversions/Clutch_Conversions/Override Checksum [0-255] ==
  note: This subsystem is used to override the model value of a signal to a constant value
  note: Override Switch Subsystem
  In1 : Inport
  Multiport Switch : MultiPortSwitch  DataPortOrder=Zero-based contiguous  Inputs=2  zeroidx=on
  Override Value : Constant  Value=0  OutDataTypeStr=double
  Signal Override Switch 0 = Use Model 1 = Use Constant : Constant  Value=0
  Out1 : Outport
  wires:
  Signal Override Switch 0 = Use Model 1 = Use Constant/1 -> Multiport Switch/1
  In1/1 -> Multiport Switch/2
  Multiport Switch/1 -> Out1/1
  Override Value/1 -> Multiport Switch/3

== system Clutch_TestBench/Camaro Fault Detection/Input Conversions/Clutch_Conversions/Override Error CAN [0-1] ==
  note: Override Switch Subsystem
  note: This subsystem is used to override the model value of a signal to a constant value
  In1 : Inport
  Multiport Switch : MultiPortSwitch  DataPortOrder=Zero-based contiguous  Inputs=2  zeroidx=on
  Override Value : Constant  OutDataTypeStr=double
  Signal Override Switch 0 = Use Model 1 = Use Constant : Constant  Value=0
  Out1 : Outport
  wires:
  Override Value/1 -> Multiport Switch/3
  Multiport Switch/1 -> Out1/1
  In1/1 -> Multiport Switch/2
  Signal Override Switch 0 = Use Model 1 = Use Constant/1 -> Multiport Switch/1

== system Clutch_TestBench/Camaro Fault Detection/Input Conversions/Clutch_Conversions/Override Error Hardware [0-1] ==
  note: This subsystem is used to override the model value of a signal to a constant value
  note: Override Switch Subsystem
  In1 : Inport
  Multiport Switch : MultiPortSwitch  DataPortOrder=Zero-based contiguous  Inputs=2  zeroidx=on
  Override Value : Constant  OutDataTypeStr=double
  Signal Override Switch 0 = Use Model 1 = Use Constant : Constant  Value=0
  Out1 : Outport
  wires:
  Signal Override Switch 0 = Use Model 1 = Use Constant/1 -> Multiport Switch/1
  In1/1 -> Multiport Switch/2
  Multiport Switch/1 -> Out1/1
  Override Value/1 -> Multiport Switch/3

== system Clutch_TestBench/Camaro Fault Detection/Input Conversions/Clutch_Conversions/Override Error Mechanical [0-1] ==
  note: Override Switch Subsystem
  note: This subsystem is used to override the model value of a signal to a constant value
  In1 : Inport
  Multiport Switch : MultiPortSwitch  DataPortOrder=Zero-based contiguous  Inputs=2  zeroidx=on
  Override Value : Constant  OutDataTypeStr=double
  Signal Override Switch 0 = Use Model 1 = Use Constant : Constant  Value=0
  Out1 : Outport
  wires:
  Override Value/1 -> Multiport Switch/3
  Multiport Switch/1 -> Out1/1
  In1/1 -> Multiport Switch/2
  Signal Override Switch 0 = Use Model 1 = Use Constant/1 -> Multiport Switch/1

== system Clutch_TestBench/Camaro Fault Detection/Input Conversions/Clutch_Conversions/Override Mode [0-7] ==
  note: Override Switch Subsystem
  note: This subsystem is used to override the model value of a signal to a constant value
  In1 : Inport
  Multiport Switch : MultiPortSwitch  DataPortOrder=Zero-based contiguous  Inputs=2  zeroidx=on
  Override Value : Constant  Value=0  OutDataTypeStr=double
  Signal Override Switch 0 = Use Model 1 = Use Constant : Constant  Value=0
  Out1 : Outport
  wires:
  Override Value/1 -> Multiport Switch/3
  Multiport Switch/1 -> Out1/1
  In1/1 -> Multiport Switch/2
  Signal Override Switch 0 = Use Model 1 = Use Constant/1 -> Multiport Switch/1

== system Clutch_TestBench/Camaro Fault Detection/Input Conversions/Clutch_Conversions/Override Position [deg] ==
  note: This subsystem is used to override the model value of a signal to a constant value
  note: Override Switch Subsystem
  In1 : Inport
  Multiport Switch : MultiPortSwitch  DataPortOrder=Zero-based contiguous  Inputs=2  zeroidx=on
  Override Value : Constant  Value=0  OutDataTypeStr=double
  Signal Override Switch 0 = Use Model 1 = Use Constant : Constant  Value=0
  Out1 : Outport
  wires:
  Signal Override Switch 0 = Use Model 1 = Use Constant/1 -> Multiport Switch/1
  In1/1 -> Multiport Switch/2
  Multiport Switch/1 -> Out1/1
  Override Value/1 -> Multiport Switch/3

== system Clutch_TestBench/Camaro Fault Detection/Input Conversions/Clutch_Conversions/Override Pressure [bar] ==
  note: Override Switch Subsystem
  note: This subsystem is used to override the model value of a signal to a constant value
  In1 : Inport
  Multiport Switch : MultiPortSwitch  DataPortOrder=Zero-based contiguous  Inputs=2  zeroidx=on
  Override Value : Constant  Value=0  OutDataTypeStr=double
  Signal Override Switch 0 = Use Model 1 = Use Constant : Constant  Value=0
  Out1 : Outport
  wires:
  Override Value/1 -> Multiport Switch/3
  Multiport Switch/1 -> Out1/1
  In1/1 -> Multiport Switch/2
  Signal Override Switch 0 = Use Model 1 = Use Constant/1 -> Multiport Switch/1

== system Clutch_TestBench/Camaro Fault Detection/Input Conversions/Clutch_Conversions/Override Temp Error [0-1] ==
  note: Override Switch Subsystem
  note: This subsystem is used to override the model value of a signal to a constant value
  In1 : Inport
  Multiport Switch : MultiPortSwitch  DataPortOrder=Zero-based contiguous  Inputs=2  zeroidx=on
  Override Value : Constant  Value=0  OutDataTypeStr=double
  Signal Override Switch 0 = Use Model 1 = Use Constant : Constant  Value=0
  Out1 : Outport
  wires:
  Override Value/1 -> Multiport Switch/3
  Multiport Switch/1 -> Out1/1
  In1/1 -> Multiport Switch/2
  Signal Override Switch 0 = Use Model 1 = Use Constant/1 -> Multiport Switch/1

== system Clutch_TestBench/Camaro Fault Detection/Input Conversions/Clutch_Conversions/Override Temp Warning [0-1] ==
  note: This subsystem is used to override the model value of a signal to a constant value
  note: Override Switch Subsystem
  In1 : Inport
  Multiport Switch : MultiPortSwitch  DataPortOrder=Zero-based contiguous  Inputs=2  zeroidx=on
  Override Value : Constant  Value=0  OutDataTypeStr=double
  Signal Override Switch 0 = Use Model 1 = Use Constant : Constant  Value=0
  Out1 : Outport
  wires:
  Signal Override Switch 0 = Use Model 1 = Use Constant/1 -> Multiport Switch/1
  In1/1 -> Multiport Switch/2
  Multiport Switch/1 -> Out1/1
  Override Value/1 -> Multiport Switch/3

== system Clutch_TestBench/Camaro Fault Detection/Input Conversions/Clutch_Conversions/Override Voltage Error [0-1] ==
  note: This subsystem is used to override the model value of a signal to a constant value
  note: Override Switch Subsystem
  In1 : Inport
  Multiport Switch : MultiPortSwitch  DataPortOrder=Zero-based contiguous  Inputs=2  zeroidx=on
  Override Value : Constant  Value=0  OutDataTypeStr=double
  Signal Override Switch 0 = Use Model 1 = Use Constant : Constant  Value=0
  Out1 : Outport
  wires:
  Signal Override Switch 0 = Use Model 1 = Use Constant/1 -> Multiport Switch/1
  In1/1 -> Multiport Switch/2
  Multiport Switch/1 -> Out1/1
  Override Value/1 -> Multiport Switch/3

== system Clutch_TestBench/Camaro Fault Detection/Signal Diagnostic/Clutch Signal Diagnostic/Rolling Alive Counter Detection ==
  In1 : Inport
  Chart : Stateflow chart  TreatAsAtomicUnit=on
  Constant : Constant  Value=0.01
  Data Type Conversion : DataTypeConversion  OutDataTypeStr=boolean
  Detect Change : simulink/Logic and Bit Operations/Detect Change  vinit=1  InputProcessing=Inherited  OutDataTypeStr=boolean
  Out1 : Outport
  wires:
  In1/1 -> Detect Change/1
  Detect Change/1 -> Chart/1(PulseDetect)
  Chart/1(flag) -> Data Type Conversion/1
  Constant/1 -> Chart/2(CycleTime)
  Data Type Conversion/1 -> Out1/1

== system Clutch_TestBench/Camaro Fault Detection/SystemDiag1/Combined_SystemDiagnostics/Override Combined_System Status ==
  note: Override Switch Subsystem
  note: This subsystem is used to override the model value of a signal to a constant value
  In1 : Inport
  Multiport Switch : MultiPortSwitch  DataPortOrder=Zero-based contiguous  Inputs=2  zeroidx=on
  Override Value : Constant  Value=0  OutDataTypeStr=double
  Signal Override Switch 0 = Use Model 1 = Use Constant : Constant  Value=0
  Out1 : Outport
  wires:
  Override Value/1 -> Multiport Switch/3
  Multiport Switch/1 -> Out1/1
  In1/1 -> Multiport Switch/2
  Signal Override Switch 0 = Use Model 1 = Use Constant/1 -> Multiport Switch/1

== system Clutch_TestBench/Camaro Fault Detection/SystemDiag1/eSystemDiagnostics/Override eSystem Status ==
  note: This subsystem is used to override the model value of a signal to a constant value
  note: Override Switch Subsystem
  In1 : Inport
  Multiport Switch : MultiPortSwitch  DataPortOrder=Zero-based contiguous  Inputs=2  zeroidx=on
  Override Value : Constant  Value=2  OutDataTypeStr=double
  Signal Override Switch 0 = Use Model 1 = Use Constant : Constant
  Out1 : Outport
  wires:
  Signal Override Switch 0 = Use Model 1 = Use Constant/1 -> Multiport Switch/1
  In1/1 -> Multiport Switch/2
  Multiport Switch/1 -> Out1/1
  Override Value/1 -> Multiport Switch/3

== system Clutch_TestBench/Camaro Fault Detection/SystemDiag1/iceSystemDiagnostics/Override iceSystem Status ==
  note: This subsystem is used to override the model value of a signal to a constant value
  note: Override Switch Subsystem
  In1 : Inport
  Multiport Switch : MultiPortSwitch  DataPortOrder=Zero-based contiguous  Inputs=2  zeroidx=on
  Override Value : Constant  Value=2  OutDataTypeStr=double
  Signal Override Switch 0 = Use Model 1 = Use Constant : Constant
  Out1 : Outport
  wires:
  Signal Override Switch 0 = Use Model 1 = Use Constant/1 -> Multiport Switch/1
  In1/1 -> Multiport Switch/2
  Multiport Switch/1 -> Out1/1
  Override Value/1 -> Multiport Switch/3

== stateflow chart Clutch_TestBench/Camaro Fault Detection/SystemDiag1/Combined_SystemDiagnostics/Combined_System_Diagnostics ==
  state CombinedSystem_Online
    en: Combined_SystemStatus=2
  state Combined_System_Offline
    en:Combined_SystemStatus=0
  state Combined_System_Limited
    en: Combined_SystemStatus=1
  (default) -> Combined_System_Offline
  Combined_System_Offline -> CombinedSystem_Online [order 1] : [ECM_Status==2&&Clutch_Status==1&&Driver_Input_Status==1&&TCM_Status==2&&BMS_Status==2&&MCU_Status==2]
  CombinedSystem_Online -> Combined_System_Offline [order 1] : [Clutch_Status==0||ECM_Status==0||Driver_Input_Status==0||TCM_Status==0||BMS_Status==0||MCU_Status==0]
  Combined_System_Limited -> CombinedSystem_Online [order 2] : [ECM_Status==2&&Clutch_Status==1&&Driver_Input_Status==1&&TCM_Status==2&&BMS_Status==2&&MCU_Status==2]
  CombinedSystem_Online -> Combined_System_Limited [order 2] : [Driver_Input_Status==1&&Clutch_Status==1&&[ECM_Status==1||TCM_Status==1||BMS_Status==1||MCU_Status==1]]
  Combined_System_Limited -> Combined_System_Offline [order 1] : [Clutch_Status==0||ECM_Status==0||Driver_Input_Status==0||TCM_Status==0||BMS_Status==0||MCU_Status==0]
  Combined_System_Offline -> Combined_System_Limited [order 2] : [Driver_Input_Status==1&&Clutch_Status==1&&[ECM_Status==1||TCM_Status==1||BMS_Status==1||MCU_Status==1]]
  data: Driver_Input_Status input; BMS_Status input; MCU_Status input; ECM_Status input; TCM_Status input; Clutch_Status input; Combined_SystemStatus output

== stateflow chart Clutch_TestBench/Camaro Fault Detection/SystemDiag1/eSystemDiagnostics/eSystem_Diagnostics ==
  state eSystem_Offline
    en:eSystemStatus=0;
  state eSystem_Online
    en: eSystemStatus=2;
  state eSystem_Limited
    en: eSystemStatus=1;
  (default) -> eSystem_Offline
  eSystem_Offline -> eSystem_Online [order 1] : [BMS_Status==2&&MCU_Status==2&&Driver_Input_Status==1&&TCM_Status==2]
  eSystem_Online -> eSystem_Offline [order 1] : [BMS_Status==0||MCU_Status==0||Driver_Input_Status==0||TCM_Status==0]
  eSystem_Limited -> eSystem_Online [order 2] : [BMS_Status==2&&...
      | MCU_Status==2&&...
      | Driver_Input_Status==1&&TCM_Status==2]
  eSystem_Online -> eSystem_Limited [order 2] : [Driver_Input_Status==1&&...
      | [BMS_Status==1||MCU_Status==1||...
      | TCM_Status==1]]
  eSystem_Limited -> eSystem_Offline [order 1] : [BMS_Status==0||...
      | MCU_Status==0||...
      | Driver_Input_Status==0||...
      | TCM_Status==0]
  eSystem_Offline -> eSystem_Limited [order 2] : [Driver_Input_Status==1&&...
      | [BMS_Status==1||MCU_Status==1||...
      | TCM_Status==1]]
  data: BMS_Status input; MCU_Status input; Driver_Input_Status input; TCM_Status input; eSystemStatus output

== stateflow chart Clutch_TestBench/Camaro Fault Detection/SystemDiag1/iceSystemDiagnostics/iceSystem_Diagnostics ==
  state iceSystem_Online
    en: iceSystemStatus=2;
  state iceSystem_Offline
    en:iceSystemStatus=0;
  state iceSystem_Limited
    en: iceSystemStatus=1;
  (default) -> iceSystem_Offline
  iceSystem_Offline -> iceSystem_Online [order 1] : [ECM_Status==2&&Clutch_Status==1&&Driver_Input_Status==1&&TCM_Status==2]
  iceSystem_Online -> iceSystem_Offline [order 1] : [ECM_Status==0||Clutch_Status==0||Driver_Input_Status==0||TCM_Status==0]
  iceSystem_Limited -> iceSystem_Online [order 2] : [ECM_Status==2&&...
      | Clutch_Status==1&&...
      | Driver_Input_Status==1&&TCM_Status==2]
  iceSystem_Online -> iceSystem_Limited [order 2] : [Driver_Input_Status==1&&...
      | Clutch_Status==1&&...
      | [ECM_Status==1||TCM_Status==1]]
  iceSystem_Limited -> iceSystem_Offline [order 1] : [ECM_Status==0||...
      | Clutch_Status==0||...
      | Driver_Input_Status==0||...
      | TCM_Status==0]
  iceSystem_Offline -> iceSystem_Limited [order 2] : [Driver_Input_Status==1&&...
      | Clutch_Status==1&&...
      | (ECM_Status==1||TCM_Status==1)]
  data: ECM_Status input; Clutch_Status input; TCM_Status input; Driver_Input_Status input; iceSystemStatus output

== stateflow chart Clutch_TestBench/Camaro Fault Detection/Signal Diagnostic/Clutch Signal Diagnostic/Rolling Alive Counter Detection/Chart ==
  state Off
    en:flag=0;
  state Alive
    en:flag=1;
  state Dead
    en:flag=0;
  Alive -> Alive [order 1] : after(CycleTime-tloop,sec)
      | [PulseDetect==1]
  (default) -> Off
  Off -> Alive : [PulseDetect==1]
  Alive -> Dead [order 2] : after(CycleTime,sec)
  data: PulseDetect input; CycleTime input; flag output; tloop parameter

== stateflow chart Clutch_TestBench/Camaro Fault Detection/Component Diagnostic/Clutch Component Diagnostic/Clutch_Comp_Diag ==
  state Clutch_Input_Offline
    en: Clutch_Status=0;
  state Clutch_Input_Online
    en: Clutch_Status=1;
  (default) -> Clutch_Input_Offline
  Clutch_Input_Online -> Clutch_Input_Offline : [Online_to_Offline==1]
  Clutch_Input_Offline -> Clutch_Input_Online : [Offline_to_Online==1]
  data: Offline_to_Online input; Online_to_Offline input; Clutch_Status output
